simulink model "sistema"  (R2021a)
settings: Solver=VariableStepAuto  StartTime=0.0  StopTime=0  RelTol=1e-3
libraries: rftxlines1 x6, rfports1 x2, rfamplifiers1 x1
settings Model: Creator=fedef  LastModifiedBy=fedef

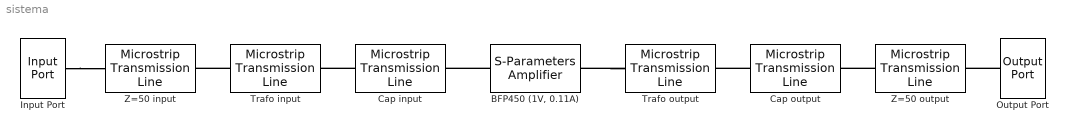
== system sistema ==
  "BFP450 (1V, 0.11A)" : rfamplifiers1/S-Parameters Amplifier  LConnTagsString=__newl0  RConnTagsString=__newr0  NetParamData=[-0.71+0.35i,0.04+0.06i;1.64+2.61i,-0.58+0.21i]  NetParamFreq=1.8e9  Z0=50  InterpMethod=Linear  IP3Type=OIP3  IIP3=inf  OIP3=inf  P1dB=inf  PSat=inf  GCSat=3  NonlinearDataFreq=2.0e9  NoiseDefinedBy=Noise figure  NF=0  FMIN=0  GammaOpt=1+0i  RN=1  NFactor=1  NTemp=0  NoiseDataFreq=2.0e9  PlotFreq=Derived from Input Port parameters  SourceFreq=Same as the s-parameters frequency  Freq=[1.9e9:1.0e8:2.2e9]  SourcePin=Extracted from data source  Pin=0  AllPlotType=X-Y plane  AppliedNetworkData=S11  AppliedComplexFormat=Magnitude (decibels)  AppliedNetworkData2=""  AppliedXParameter=Freq  YOption=Linear  XOption=Linear  PlotZ0=50  PlotFreqNoSim=User-specified  DisplayData=off  NetworkData=S11  SmithData=S11  PolarData=S11  ComplexFormat=Magnitude (decibels)  DBFormat=Magnitude (decibels)  NoneFormat=None
      settings: SourceProductBaseCode=RB
  Cap input : rftxlines1/Microstrip Transmission Line  LConnTagsString=__newl0  RConnTagsString=__newr0  Width=7.29e-3  Height=1.6e-3  Thickness=35e-6  EpsilonR=4.15  LossTangent=0  SigmaCond=inf  LineLength=19.38e-3  StubMode=Shunt  Termination=Open  PlotFreq=User-specified  SourceFreq=User-specified  Freq=[1e9:1.0e6:3e9]  AllPlotType=X-Y plane  AppliedNetworkData=S21  AppliedComplexFormat=Angle (degrees)  AppliedNetworkData2=S11  AppliedComplexFormat2=dB  AppliedXParameter=Freq  YOption=Linear  XOption=Linear  PlotZ0=50  DisplayData=off  PlotFreqNoSim=User-specified  NetworkData=S21  SmithData=S11  PolarData=S11  ComplexFormat=Angle  DBFormat=Magnitude (decibels)  NoneFormat=None
      settings: SourceProductBaseCode=RB
  Cap output : rftxlines1/Microstrip Transmission Line  LConnTagsString=__newl0  RConnTagsString=__newr0  Width=4.99e-3  Height=1.6e-3  Thickness=35e-6  EpsilonR=4.15  LossTangent=0  SigmaCond=inf  LineLength=0.01  StubMode=Shunt  Termination=Open  PlotFreq=User-specified  SourceFreq=User-specified  Freq=[1e9:1.0e6:3e9]  AllPlotType=X-Y plane  AppliedNetworkData=S21  AppliedComplexFormat=Angle (degrees)  AppliedNetworkData2=S11  AppliedComplexFormat2=dB  AppliedXParameter=Freq  YOption=Linear  XOption=Linear  PlotZ0=50  DisplayData=off  PlotFreqNoSim=User-specified  NetworkData=S21  SmithData=S11  PolarData=S11  ComplexFormat=Angle  DBFormat=Magnitude (decibels)  NoneFormat=None
      settings: SourceProductBaseCode=RB
  Input Port : rfports1/Input Port  Description=source block  TreatSimulinkInputSignalAs=Incident power wave  MaxLength=128  FracBW=0  ModelDelay=0  Fc=1.8e9  Ts=1e-7  Zs=50  RFhasDSP=Elements as channels (sample based)  NoiseFlag=on  seed=67987  GoToTag=RFTag
      settings: SourceProductBaseCode=RB
  Output Port : rfports1/Output Port  Zl=50  Flag=0  num_Models=0  GoToTag=RFTag  PlotFreq=User-specified  SourceFreq=Derived from Input Port parameters  Freq=1e9:1e8:3e9  AllPlotType=X-Y plane  AppliedNetworkData=S11  AppliedComplexFormat=Magnitude (decibels)  AppliedNetworkData2=""  AppliedXParameter=Freq  AppliedXFormat=Hz  YOption=Linear  XOption=Linear  PlotZ0=50  DisplayData=off  NoBudgetPlot=Composite data  NetworkData=S11  SmithData=S11  PolarData=S11  ComplexFormat=Magnitude (decibels)  DBFormat=Magnitude (decibels)  DBMFormat=dBm  NoneFormat=None
      settings: SourceProductBaseCode=RB
  Trafo input : rftxlines1/Microstrip Transmission Line  LConnTagsString=__newl0  RConnTagsString=__newr0  Width=7.29e-3  Height=1.6e-3  Thickness=35e-6  EpsilonR=4.15  LossTangent=0  SigmaCond=inf  LineLength=22.59e-3  StubMode=Not a stub  Termination=Open  PlotFreq=User-specified  SourceFreq=User-specified  Freq=[1e9:1.0e6:3e9]  AllPlotType=X-Y plane  AppliedNetworkData=S21  AppliedComplexFormat=Angle (degrees)  AppliedNetworkData2=""  AppliedXParameter=Freq  YOption=Linear  XOption=Linear  PlotZ0=50  DisplayData=off  PlotFreqNoSim=User-specified  NetworkData=S21  SmithData=S11  PolarData=S11  ComplexFormat=Angle  DBFormat=Magnitude (decibels)  NoneFormat=None
      settings: SourceProductBaseCode=RB
  Trafo output : rftxlines1/Microstrip Transmission Line  LConnTagsString=__newl0  RConnTagsString=__newr0  Width=5.99e-3  Height=1.6e-3  Thickness=35e-6  EpsilonR=4.15  LossTangent=0  SigmaCond=inf  LineLength=22.7e-3  StubMode=Not a stub  Termination=Open  PlotFreq=User-specified  SourceFreq=User-specified  Freq=[1e9:1.0e6:3e9]  AllPlotType=X-Y plane  AppliedNetworkData=S21  AppliedComplexFormat=Angle (degrees)  AppliedNetworkData2=""  AppliedXParameter=Freq  YOption=Linear  XOption=Linear  PlotZ0=50  DisplayData=off  PlotFreqNoSim=User-specified  NetworkData=S21  SmithData=S11  PolarData=S11  ComplexFormat=Angle  DBFormat=Magnitude (decibels)  NoneFormat=None
      settings: SourceProductBaseCode=RB
  Z=50 input : rftxlines1/Microstrip Transmission Line  LConnTagsString=__newl0  RConnTagsString=__newr0  Width=3.19e-3  Height=1.6e-3  Thickness=35e-6  EpsilonR=4.15  LossTangent=0  SigmaCond=inf  LineLength=0.01  StubMode=Not a stub  Termination=Open  PlotFreq=User-specified  SourceFreq=User-specified  Freq=[1e9:1.0e6:3e9]  AllPlotType=X-Y plane  AppliedNetworkData=S21  AppliedComplexFormat=Angle (degrees)  AppliedNetworkData2=""  AppliedXParameter=Freq  YOption=Linear  XOption=Log  PlotZ0=50  DisplayData=off  PlotFreqNoSim=User-specified  NetworkData=S21  SmithData=S11  PolarData=S11  ComplexFormat=Angle  DBFormat=Magnitude (decibels)  NoneFormat=None
      settings: SourceProductBaseCode=RB
  Z=50 output : rftxlines1/Microstrip Transmission Line  LConnTagsString=__newl0  RConnTagsString=__newr0  Width=3.19e-3  Height=1.6e-3  Thickness=35e-6  EpsilonR=4.15  LossTangent=0  SigmaCond=inf  LineLength=0.01  StubMode=Not a stub  Termination=Open  PlotFreq=User-specified  SourceFreq=User-specified  Freq=[1e9:1.0e6:3e9]  AllPlotType=X-Y plane  AppliedNetworkData=S21  AppliedComplexFormat=Angle (degrees)  AppliedNetworkData2=""  AppliedXParameter=Freq  YOption=Linear  XOption=Log  PlotZ0=50  DisplayData=off  PlotFreqNoSim=User-specified  NetworkData=S21  SmithData=S11  PolarData=S11  ComplexFormat=Angle  DBFormat=Magnitude (decibels)  NoneFormat=None
      settings: SourceProductBaseCode=RB
  connections:
  Trafo input/LConn1 -- Z=50 input/RConn1
  Cap input/LConn1 -- Trafo input/RConn1
  "BFP450 (1V, 0.11A)"/LConn1 -- Cap input/RConn1
  Trafo output/LConn1 -- "BFP450 (1V, 0.11A)"/RConn1
  Cap output/LConn1 -- Trafo output/RConn1
  Z=50 output/LConn1 -- Cap output/RConn1
  Input Port/RConn1 -- Z=50 input/LConn1
  Output Port/LConn1 -- Z=50 output/RConn1
